simulink model "control"  (R2024b)
settings: Solver=VariableStepAuto  StartTime=0.0  StopTime=4  RelTol=1e-3
values from neighbouring files (symbols this model uses):
  Tc = 0.001    [generated traj.mat]
undefined symbols (not defined in the file or in its folder): DiscIntNeverNeededParam
settings Model: Creator=giuseppeloianno  LastModifiedBy=22guo
settings OptimizationCC: ReuseModelBlockBuffer=off
settings RTWCC: GPUComputeCapability=3.5

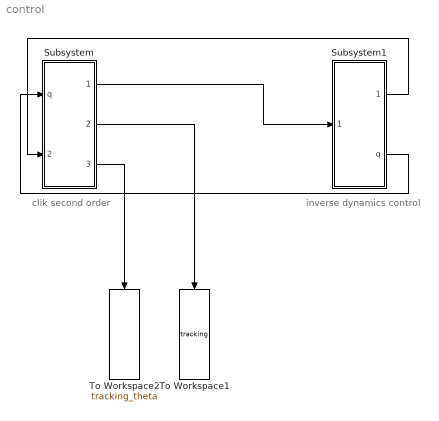
== system control ==
  note: clik second order
  note: inverse dynamics control
  Subsystem : Subsystem
  Subsystem1 : Subsystem
  To Workspace1 : ToWorkspace  VariableName=tracking  SampleTime=-1
      settings: Save2DSignal=2-D array (concatenate along first dimension)
  To Workspace2 : ToWorkspace  VariableName=tracking_theta  SampleTime=-1
      settings: Save2DSignal=2-D array (concatenate along first dimension)
  wires:
  Subsystem/1(q_dot_dot) -> Subsystem1/1(q_dot_dot)
  Subsystem/3(Out1) -> To Workspace2/1
  Subsystem/2(Out3) -> To Workspace1/1
  Subsystem1/2(q) -> Subsystem/1(q)
  Subsystem1/1(q_dot) -> Subsystem/2(q_dot)

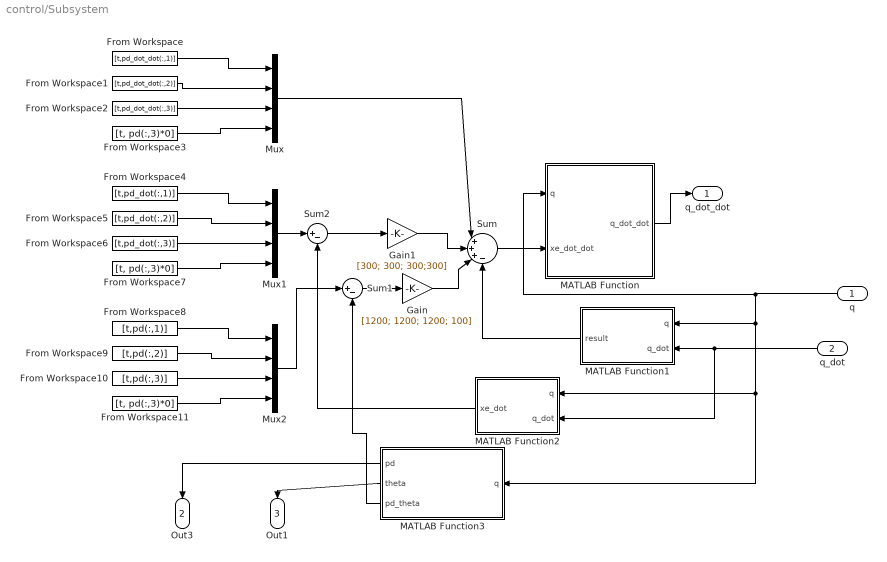
== system control/Subsystem ==
  q : Inport
  q_dot : Inport  Port=2
  From Workspace : FromWorkspace  VariableName=[t,pd_dot_dot(:,1)]  SampleTime=Tc
  From Workspace1 : FromWorkspace  VariableName=[t,pd_dot_dot(:,2)]  SampleTime=Tc
  From Workspace10 : FromWorkspace  VariableName=[t,pd(:,3)]  SampleTime=0.001
  From Workspace11 : FromWorkspace  VariableName=[t, pd(:,3)*0]  SampleTime=0.001
  From Workspace2 : FromWorkspace  VariableName=[t,pd_dot_dot(:,3)]  SampleTime=Tc
  From Workspace3 : FromWorkspace  VariableName=[t, pd(:,3)*0]  SampleTime=Tc
  From Workspace4 : FromWorkspace  VariableName=[t,pd_dot(:,1)]  SampleTime=Tc
  From Workspace5 : FromWorkspace  VariableName=[t,pd_dot(:,2)]  SampleTime=Tc
  From Workspace6 : FromWorkspace  VariableName=[t,pd_dot(:,3)]  SampleTime=Tc
  From Workspace7 : FromWorkspace  VariableName=[t, pd(:,3)*0]  SampleTime=Tc
  From Workspace8 : FromWorkspace  VariableName=[t,pd(:,1)]  SampleTime=0.001
  From Workspace9 : FromWorkspace  VariableName=[t,pd(:,2)]  SampleTime=0.001
  Gain : Gain  Gain=[1200; 1200; 1200; 100]
  Gain1 : Gain  Gain=[300; 300; 300;300]
  MATLAB Function : MATLAB Function  TreatAsAtomicUnit=on
  MATLAB Function1 : MATLAB Function  TreatAsAtomicUnit=on
  MATLAB Function2 : MATLAB Function  TreatAsAtomicUnit=on
  MATLAB Function3 : MATLAB Function  TreatAsAtomicUnit=on
  Mux : Mux
  Mux1 : Mux
  Mux2 : Mux
  Sum : Sum  Inputs=|+++-
  Sum1 : Sum  Inputs=|+-
  Sum2 : Sum  Inputs=|+-
  q_dot_dot : Outport
  Out3 : Outport  Port=2
  Out1 : Outport  Port=3
  wires:
  From Workspace/1 -> Mux/1
  MATLAB Function2/1(xe_dot) -> Sum2/2
  From Workspace4/1 -> Mux1/1
  MATLAB Function3/1(pd) -> Out3/1
  From Workspace5/1 -> Mux1/2
  Mux1/1 -> Sum2/1
  From Workspace11/1 -> Mux2/4
  Sum1/1 -> Gain/1
  From Workspace2/1 -> Mux/3
  From Workspace7/1 -> Mux1/4
  Gain/1 -> Sum/3
  Sum2/1 -> Gain1/1
  Mux/1 -> Sum/1
  From Workspace6/1 -> Mux1/3
  From Workspace1/1 -> Mux/2
  From Workspace9/1 -> Mux2/2
  From Workspace10/1 -> Mux2/3
  MATLAB Function3/2(theta) -> Out1/1
  Mux2/1 -> Sum1/1
  Sum/1 -> MATLAB Function/2(xe_dot_dot)
  Gain1/1 -> Sum/2
  MATLAB Function3/3(pd_theta) -> Sum1/2
  From Workspace3/1 -> Mux/4
  From Workspace8/1 -> Mux2/1
  MATLAB Function/1(q_dot_dot) -> q_dot_dot/1
  q/1 -> MATLAB Function/1(q), MATLAB Function3/1(q), MATLAB Function2/1(q), MATLAB Function1/1(q)
  q_dot/1 -> MATLAB Function2/2(q_dot), MATLAB Function1/2(q_dot)
  MATLAB Function1/1(result) -> Sum/4

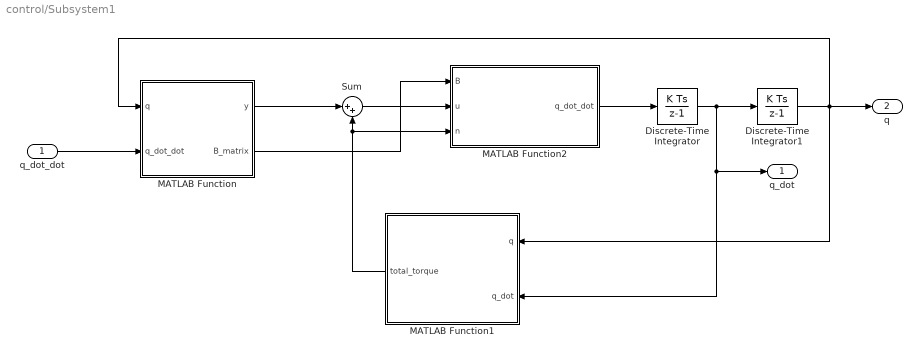
== system control/Subsystem1 ==
  q_dot_dot : Inport
  Discrete-Time Integrator : DiscreteIntegrator  InitialCondition=[0; 0; 0; 0]  SampleTime=0.001  ICPrevOutput=DiscIntNeverNeededParam  ICPrevScaledInput=DiscIntNeverNeededParam
  Discrete-Time Integrator1 : DiscreteIntegrator  InitialCondition=[0.7; 0.5; 0.5; 0]  SampleTime=-1  ICPrevOutput=DiscIntNeverNeededParam  ICPrevScaledInput=DiscIntNeverNeededParam
  MATLAB Function : MATLAB Function  TreatAsAtomicUnit=on
  MATLAB Function1 : MATLAB Function  TreatAsAtomicUnit=on
  MATLAB Function2 : MATLAB Function  TreatAsAtomicUnit=on
  Sum : Sum  Inputs=|++
  q_dot : Outport
  q : Outport  Port=2
  wires:
  Discrete-Time Integrator/1 -> Discrete-Time Integrator1/1, MATLAB Function1/2(q_dot), q_dot/1
  Discrete-Time Integrator1/1 -> MATLAB Function/1(q), q/1, MATLAB Function1/1(q)
  MATLAB Function/1(y) -> Sum/1
  MATLAB Function1/1(total_torque) -> MATLAB Function2/3(n), Sum/2
  MATLAB Function2/1(q_dot_dot) -> Discrete-Time Integrator/1
  Sum/1 -> MATLAB Function2/2(u)
  MATLAB Function/2(B_matrix) -> MATLAB Function2/1(B)
  q_dot_dot/1 -> MATLAB Function/2(q_dot_dot)

== matlab function control/Subsystem/MATLAB Function ==
  data: q input; xe_dot_dot input; q_dot_dot output
function q_dot_dot = J_Inverse(q,xe_dot_dot)
[q_dot_dot] = jacobian_inverse(q, xe_dot_dot);
end

== matlab function control/Subsystem/MATLAB Function2 ==
  data: q input; xe_dot output; q_dot input
function xe_dot = Jacobian(q,q_dot)
xe_dot=jacobian(q,q_dot);
end

== matlab function control/Subsystem/MATLAB Function3 ==
  data: q input; pd output; theta output; pd_theta output
function [pd,theta,pd_theta] = direct_kin(q)
[pd, theta, pd_theta]= direct_kin(q);
end

== matlab function control/Subsystem1/MATLAB Function ==
  data: q input; y output; B_matrix output; q_dot_dot input
function [y,B_matrix] = B(q,q_dot_dot)
[y,B_matrix]=B(q,q_dot_dot);
end

== matlab function control/Subsystem1/MATLAB Function1 ==
  data: q input; total_torque output; q_dot input
function total_torque = n(q, q_dot)

total_torque=n(q,q_dot);
end

== matlab function control/Subsystem1/MATLAB Function2 ==
  data: B input; u input; q_dot_dot output; n input
function q_dot_dot = Manipulator(B,u,n)

q_dot_dot=manipulator(B,u,n);

end

== matlab function control/Subsystem/MATLAB Function1 ==
  data: q input; result output; q_dot input
function result = J_dot(q,q_dot)
 result = jacobian_dot(q,q_dot);
end
